simulink model "PolynomialController"  (R2021a)
settings: Solver=FixedStepAuto  StartTime=0.0  StopTime=SimTime-Ts  FixedStep=1e-3  RelTol=1e-3
values from neighbouring files (symbols this model uses):
  C12 = x(3)    [DigitalPIDRunner.m]    (also in DoubleMassRunner.m; NNIdentify.m = Xnt_noise(3); NNTrainingSet.m = T(i, 3); PIDModalController.m = 16.6338)
  k1 = x(1)    [DigitalPIDRunner.m]    (also in DoubleMassRunner.m; NNIdentify.m = Xnt_noise(1); NNTrainingSet.m = T(i, 1); PIDModalController.m = 0.2244)
  k2 = x(2)    [DigitalPIDRunner.m]    (also in DoubleMassRunner.m; NNIdentify.m = Xnt_noise(2); NNTrainingSet.m = T(i, 2); PIDModalController.m = 0.5636)
  Ts = 1e-3    (= 0.001)    [DigitalPIDRunner.m]    (also in DoubleMassRunner.m = ref.Ts; NNTrainingSet.m; PIDModalController.m; PIDRunner.m = p.Results.StepTime)
undefined symbols (not defined in the file or in its folder): C_poly, r0, R_poly
settings Model: Creator=akangmufti  LastModifiedBy=akangmufti

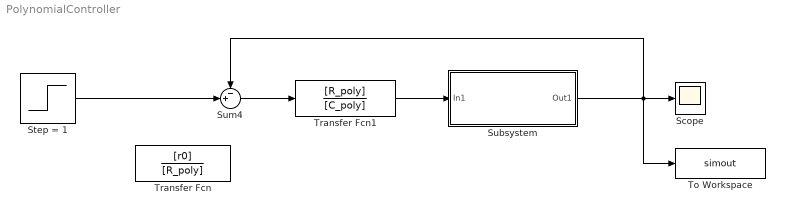
== system PolynomialController ==
  Scope : Scope
  Step = 1 : Step  Time=0.0001  SampleTime=0
  Subsystem : Subsystem
  Sum4 : Sum  Inputs=-+|
  To Workspace : ToWorkspace  VariableName=simout  SampleTime=Ts
      settings: Save2DSignal=2-D array (concatenate along first dimension)
  Transfer Fcn : TransferFcn  Numerator=[r0]  Denominator=[R_poly]
  Transfer Fcn1 : TransferFcn  Numerator=[R_poly]  Denominator=[C_poly]
  wires:
  Sum4/1 -> Transfer Fcn1/1
  Transfer Fcn1/1 -> Subsystem/1(In1)
  Subsystem/1(Out1) -> Sum4/1, Scope/1, To Workspace/1
  Step = 1/1 -> Sum4/2

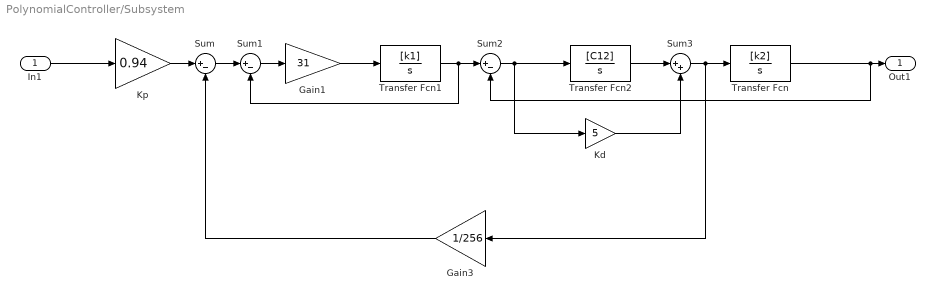
== system PolynomialController/Subsystem ==
  In1 : Inport
  Gain1 : Gain  Gain=31
  Gain3 : Gain  Gain=1/256
  Kd : Gain  Gain=5
  Kp : Gain  Gain=0.94
  Sum : Sum  Inputs=|+-
  Sum1 : Sum  Inputs=|+-
  Sum2 : Sum  Inputs=|+-
  Sum3 : Sum  Inputs=|++
  Transfer Fcn : TransferFcn  Numerator=[k2]  Denominator=[1 0]
  Transfer Fcn1 : TransferFcn  Numerator=[k1]  Denominator=[1 0]
  Transfer Fcn2 : TransferFcn  Numerator=[C12]  Denominator=[1 0]
  Out1 : Outport
  wires:
  Kp/1 -> Sum/1
  Transfer Fcn1/1 -> Sum2/1, Sum1/2
  Gain1/1 -> Transfer Fcn1/1
  Sum2/1 -> Kd/1, Transfer Fcn2/1
  Sum1/1 -> Gain1/1
  Gain3/1 -> Sum/2
  Sum/1 -> Sum1/1
  Sum3/1 -> Transfer Fcn/1, Gain3/1
  Transfer Fcn2/1 -> Sum3/1
  In1/1 -> Kp/1
  Kd/1 -> Sum3/2
  Transfer Fcn/1 -> Sum2/2, Out1/1
